simulink model "experiment201"  (R2018b)
settings: Solver=VariableStepAuto  StartTime=0.0  StopTime=10.0  RelTol=1e-3
settings Model: Creator=HIT-QJ  LastModifiedBy=HIT-QJ

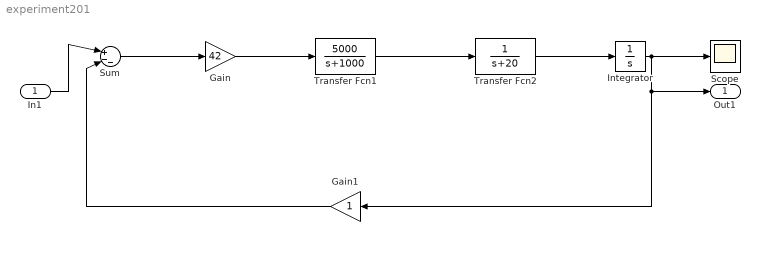
== system experiment201 ==
  In1 : Inport
  Gain : Gain  Gain=42
  Gain1 : Gain
  Integrator : Integrator
  Scope : Scope
  Sum : Sum  Inputs=|+--
  Transfer Fcn1 : TransferFcn  Numerator=[5000]  Denominator=[1 1000]
  Transfer Fcn2 : TransferFcn  Denominator=[1 20]
  Out1 : Outport
  wires:
  In1/1 -> Sum/1
  Sum/1 -> Gain/1
  Gain/1 -> Transfer Fcn1/1
  Transfer Fcn1/1 -> Transfer Fcn2/1
  Transfer Fcn2/1 -> Integrator/1
  Integrator/1 -> Gain1/1, Out1/1, Scope/1
  Gain1/1 -> Sum/2
